simulink model "hardwareekf"  (R2021a)
settings: Solver=FixedStepAuto  StartTime=0.0  StopTime=2  FixedStep=0.5  RelTol=1e-3
undefined symbols (not defined in the file or in its folder): DiscIntNeverNeededParam
libraries: simulink x3
settings Model: Creator=ACER  LastModifiedBy=ACER

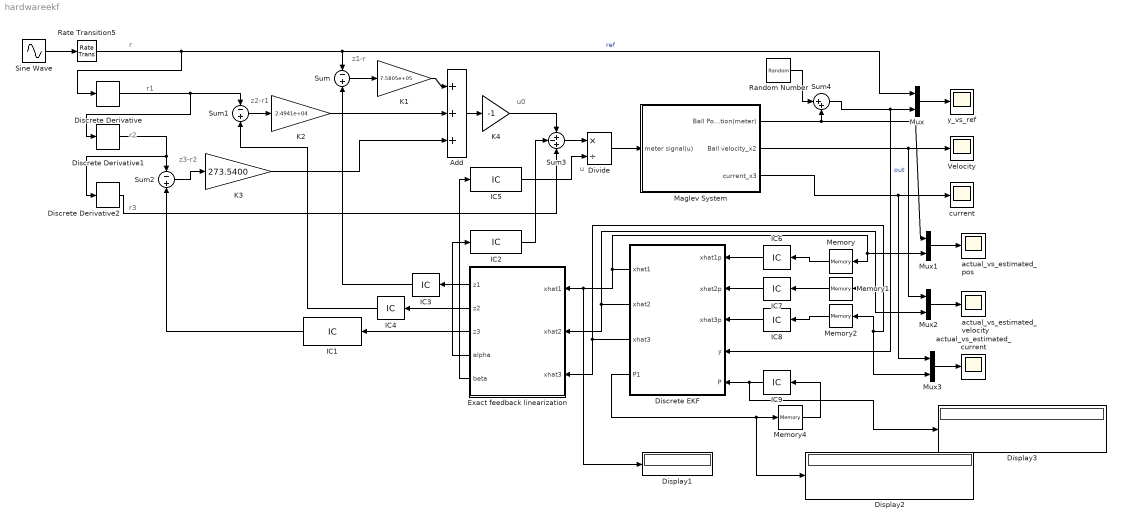
== system hardwareekf ==
  note: u0
  note: z3-r2
  note: z2-r1
  note: z1-r
  note: r
  note: r1
  note: r2
  note: r3
  note: u
  Add : Sum  Inputs=+++
  Discrete Derivative : simulink/Discrete/Discrete Derivative  gainval=1.0  ICPrevScaledInput=0.0  OutMin=[]  OutMax=[]  OutDataType=fixdt(1, 16)  OutScaling=2^-10  DoSatur=off
  Discrete Derivative1 : simulink/Discrete/Discrete Derivative  gainval=1.0  ICPrevScaledInput=0.0  OutMin=[]  OutMax=[]  OutDataType=fixdt(1, 16)  OutScaling=2^-10  DoSatur=off
  Discrete Derivative2 : simulink/Discrete/Discrete Derivative  gainval=1.0  ICPrevScaledInput=0.0  OutMin=[]  OutMax=[]  OutDataType=fixdt(1, 16)  OutScaling=2^-10  DoSatur=off
  Discrete EKF : MATLAB Function  TreatAsAtomicUnit=on
  Display1 : Display
  Display2 : Display
  Display3 : Display
  Divide : Product  Inputs=*/
  "Exact feedback linearization " : MATLAB Function  TreatAsAtomicUnit=on
  IC1 : InitialCondition  Value=1.7764e-15
  IC2 : InitialCondition  Value=-102.8932
  IC3 : InitialCondition  Value=0.0095
  IC4 : InitialCondition  Value=0
  IC5 : InitialCondition  Value=1.9015e+03
  IC6 : InitialCondition  Value=0.0095
  IC7 : InitialCondition  Value=0
  IC8 : InitialCondition  Value=0.8400
  IC9 : InitialCondition  Value=[0.1 0 0;0 0.1 0;0 0 0.1]
  K1 : Gain  Gain=7.5805e+05
  K2 : Gain  Gain=2.4941e+04
  K3 : Gain  Gain=273.5400
  K4 : Gain  Gain=-1
  Maglev System : Subsystem
  Memory{,1..2,4} (4 alike) : Memory
  Mux{,1..3} (4 alike) : Mux  Inputs=2
  Random Number : RandomNumber  Variance=5e-6  SampleTime=0.5
  Rate Transition5 : RateTransition  OutPortSampleTime=0.5
  Sine Wave : Sin  SampleTime=0
  Sum : Sum  Inputs=-+
  Sum1 : Sum  Inputs=-+
  Sum2 : Sum  Inputs=-+
  Sum3 : Sum  Inputs=+-+
  Sum4 : Sum  Inputs=|++
  Velocity : Scope
  actual_vs_estimated_current : Scope
  actual_vs_estimated_pos : Scope
  actual_vs_estimated_velocity : Scope
  current : Scope
  y_vs_ref : Scope
  wires:
  "Exact feedback linearization "/1(z1) -> IC3/1
  Sum/1 -> K1/1
  "Exact feedback linearization "/2(z2) -> IC4/1
  Sum1/1 -> K2/1
  "Exact feedback linearization "/3(z3) -> IC1/1
  K1/1 -> Add/1
  K2/1 -> Add/2
  Sum2/1 -> K3/1
  K3/1 -> Add/3
  Add/1 -> K4/1
  K4/1 -> Sum3/1
  "Exact feedback linearization "/4(alpha) -> IC2/1
  Sum3/1 -> Divide/1
  "Exact feedback linearization "/5(beta) -> IC5/1
  Divide/1 -> Maglev System/1(meter signal(u))
  Maglev System/1(Ball Position(meter)) -> Mux1/1, Sum4/2
  Random Number/1 -> Sum4/1
  Mux/1 -> y_vs_ref/1
  Maglev System/2(Ball velocity_x2) -> Mux2/1, Velocity/1
  Maglev System/3(current_x3) -> Mux3/1, current/1
  Mux1/1 -> actual_vs_estimated_pos/1
  Mux2/1 -> actual_vs_estimated_velocity/1
  Mux3/1 -> actual_vs_estimated_current/1
  Sine Wave/1 -> Rate Transition5/1
  Discrete Derivative/1 -> Discrete Derivative1/1, Sum1/1
  Discrete Derivative1/1 -> Discrete Derivative2/1, Sum2/1
  Discrete Derivative2/1 -> Sum3/3
  Discrete EKF/4(P1) -> Display2/1, Memory4/1
  Sum4/1 -> Discrete EKF/4(y), Mux/2  "out"
  Memory4/1 -> IC9/1
  Rate Transition5/1 -> Discrete Derivative/1, Mux/1, Sum/1  "ref"
  Discrete EKF/1(xhat1) -> Memory/1, Mux1/2, Display1/1, "Exact feedback linearization "/1(xhat1)
  Discrete EKF/2(xhat2) -> Mux2/2, Memory1/1, "Exact feedback linearization "/2(xhat2)
  Discrete EKF/3(xhat3) -> Memory2/1, Mux3/2, "Exact feedback linearization "/3(xhat3)
  IC3/1 -> Sum/2
  IC4/1 -> Sum1/2
  IC1/1 -> Sum2/2
  IC2/1 -> Sum3/2
  IC5/1 -> Divide/2
  IC6/1 -> Discrete EKF/1(xhat1p)
  Memory/1 -> IC6/1
  IC7/1 -> Discrete EKF/2(xhat2p)
  Memory1/1 -> IC7/1
  Memory2/1 -> IC8/1
  IC8/1 -> Discrete EKF/3(xhat3p)
  IC9/1 -> Display3/1, Discrete EKF/5(P)

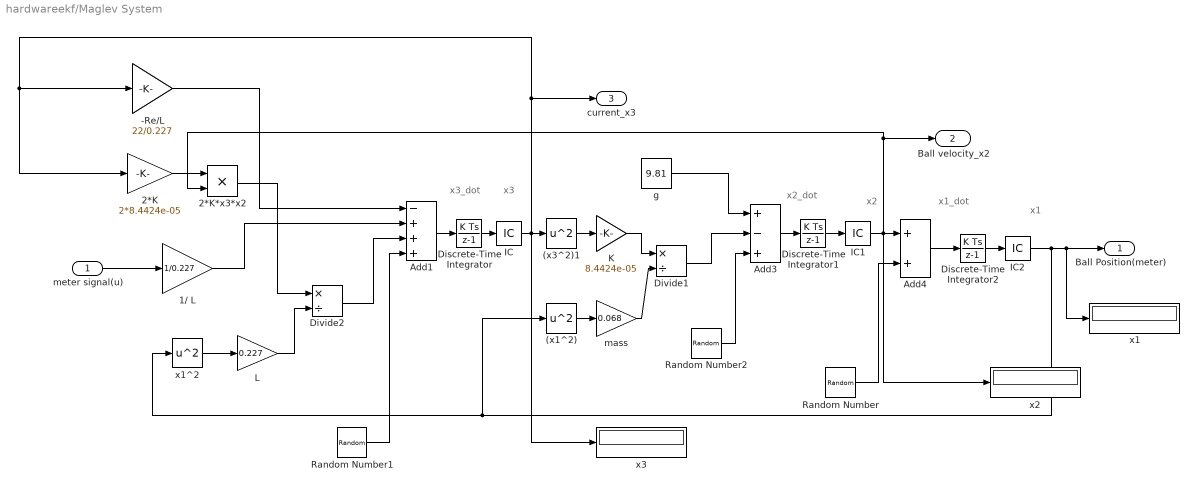
== system hardwareekf/Maglev System ==
  note: x3_dot
  note: x3
  note: x2_dot
  note: x2
  note: x1_dot
  note: x1
  meter signal(u) : Inport
  (x1^2) : Math  Operator=square  SaturateOnIntegerOverflow=on
  (x3^2)1 : Math  Operator=square  SaturateOnIntegerOverflow=on
  -Re/L : Gain  Gain=22/0.227
  1/	L : Gain  Gain=1/0.227
  2*K : Gain  Gain=2*8.4424e-05
  2*K*x3*x2 : Product
  Add1 : Sum  Inputs=-+++
  Add3 : Sum  Inputs=+-+
  Add4 : Sum
  Discrete-Time Integrator : DiscreteIntegrator  SampleTime=-1  ICPrevOutput=DiscIntNeverNeededParam  ICPrevScaledInput=DiscIntNeverNeededParam
  Discrete-Time Integrator1 : DiscreteIntegrator  SampleTime=-1  ICPrevOutput=DiscIntNeverNeededParam  ICPrevScaledInput=DiscIntNeverNeededParam
  Discrete-Time Integrator2 : DiscreteIntegrator  SampleTime=-1  ICPrevOutput=DiscIntNeverNeededParam  ICPrevScaledInput=DiscIntNeverNeededParam
  Divide1 : Product  Inputs=*/
  Divide2 : Product  Inputs=*/
  IC : InitialCondition  Value=0.8
  IC1 : InitialCondition  Value=0
  IC2 : InitialCondition  Value=0.009
  K : Gain  Gain=8.4424e-05
  L : Gain  Gain=0.227
  Random Number : RandomNumber  Variance=0.0001  SampleTime=0.5
  Random Number1 : RandomNumber  Variance=0.0001  SampleTime=0.5
  Random Number2 : RandomNumber  Variance=0.0001  SampleTime=0.5
  g : Constant  Value=9.81  SampleTime=0.5
  mass : Gain  Gain=0.068
  x1 : Display
  x1^2 : Math  Operator=square  SaturateOnIntegerOverflow=on
  x2 : Display
  x3 : Display
  Ball Position(meter) : Outport
  Ball velocity_x2 : Outport  Port=2
  current_x3 : Outport  Port=3
  wires:
  meter signal(u)/1 -> 1/	L/1
  Discrete-Time Integrator2/1 -> IC2/1
  x1^2/1 -> L/1
  Add1/1 -> Discrete-Time Integrator/1
  g/1 -> Add3/1
  Add3/1 -> Discrete-Time Integrator1/1
  Add4/1 -> Discrete-Time Integrator2/1
  2*K/1 -> 2*K*x3*x2/1
  Random Number/1 -> Add4/2
  Random Number1/1 -> Add1/4
  Random Number2/1 -> Add3/3
  (x3^2)1/1 -> K/1
  (x1^2)/1 -> mass/1
  K/1 -> Divide1/1
  mass/1 -> Divide1/2
  Divide1/1 -> Add3/2
  -Re/L/1 -> Add1/1
  1/	L/1 -> Add1/2
  Divide2/1 -> Add1/3
  L/1 -> Divide2/2
  2*K*x3*x2/1 -> Divide2/1
  Discrete-Time Integrator/1 -> IC/1
  IC/1 -> x3/1, current_x3/1, 2*K/1, -Re/L/1, (x3^2)1/1
  Discrete-Time Integrator1/1 -> IC1/1
  IC1/1 -> x2/1, 2*K*x3*x2/2, Ball velocity_x2/1, Add4/1
  IC2/1 -> (x1^2)/1, x1^2/1, x1/1, Ball Position(meter)/1

== matlab function hardwareekf/Exact feedback linearization  ==
  data: xhat1 input; z1 output; xhat2 input; xhat3 input; z2 output; z3 output; alpha output; beta output
function [z1,z2,z3,alpha,beta] = Exact_fb_linearization(xhat1,xhat2,xhat3)

x0 = 0.009;                               %initial position in meter
mass = 0.068;                            %Kg (mass of the ball))
g = 9.81;
L0 = 0.018761;                          %Henry (Kg)(m^2)(s^-2)(A^-2)
Lind=0.227;                              %Henry(in terms of x as a meter)
K = (x0*L0)/2;                          %electromagnet force constant
Re= 22;     
 z1 = xhat1;
 z2 = xhat2; % Chec once with JUST k also the previous version of program with i+1 in this step
 z3 = g-((K*xhat3)^2)/(mass*xhat1^2);
 %componets of nonlinear feedback
 alpha=(2*K*xhat3^2*xhat2)/(mass*xhat1^3)+(2*K*Re*xhat3^2)/(mass*Lind*xhat1^2)-(4*K^2*xhat3^2*xhat2)/(mass*Lind*xhat1^4);
beta=(-2*K*xhat3)/(mass*Lind*xhat1^2);

== matlab function hardwareekf/Discrete EKF ==
  data: xhat1p input; xhat1 output; xhat2p input; xhat3p input; xhat2 output; xhat3 output; P1 output; y input; P input
function [xhat1,xhat2,xhat3,P1]  = Discrete_EKF(xhat1p,xhat2p,xhat3p,y,P)
%*********Constants***********
x0 = 0.009;                               %initial position in meter
mass = 0.068;                            %Kg (mass of the ball))
L0 = 0.018761;                          %Henry (Kg)(m^2)(s^-2)(A^-2)
Lind=0.227;                              %Henry(in terms of x as a meter)
K = (x0*L0)/2 ;                         %electromagnet force constant
Re= 22;                                  %ohm
varw = [0.0001 0.0001 0.0001]';                    %nominal process noise w0(t) = 0; i=1,2,3,...
varv = [5e-6] ;
%Update the state matrix A
A21 = (2*K*(xhat3p^2))/(mass*(xhat1p^3));
A23 = (-2*K*xhat3p)/(mass*(xhat1p^2));
A31 = (-4*K*xhat3p*xhat2p)/(Lind*xhat1p^3);
A32 = (2*K*xhat3p)/(Lind*xhat1p^2);
A33 = (-Re/Lind)+((2*K*xhat2p)/(Lind*xhat1p^2));
A = [0 1 0;A21 0 A23;A31 A32 A33]
L  = eye(3);
Q = diag(varw);
R = diag(varv);
H = [1 0 0];
M = [1 0 0];
P = A*P*A' +L*Q*L'
statep = [xhat1p;xhat2p;xhat3p];
state_out = A*statep;
Kalg = P*H'/(H*P*H'+M*R*M');
state = state_out +Kalg*(y-state_out(1));
P = (eye(1)- Kalg*H)*P
xhat1 = state(1)
xhat2 = state(2)
xhat3 = state(3)
P1=P
